simulink model "lab10_3"  (R2016a)
settings: Solver=VariableStepAuto  StartTime=0.0  StopTime=10.0  RelTol=1e-3
libraries: dspsrcs4 x1
settings Model: Creator=Student  LastModifiedBy=Student

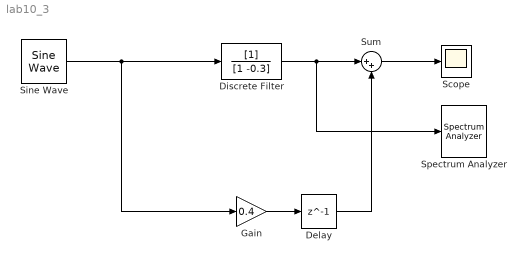
== system lab10_3 ==
  Delay : Delay  DelayLength=1  InitialCondition=0
  Discrete Filter : DiscreteFilter  Denominator=[1 -0.3]
  Gain : Gain  Gain=0.4
  Scope : Scope
  Sine Wave : dspsrcs4/Sine Wave  Amplitude=1  Frequency=100  Phase=0  SampleMode=Discrete  OutComplex=Real  CompMethod=Trigonometric fcn  TableSize=Speed  SampleTime=1/1000  SamplesPerFrame=1  ResetState=Restart at time zero  OutputFrames=off  dataType=double  wordLen=16  udDataType=sfix(16)  fracBitsMode=Best precision  numFracBits=15  OutDataTypeStr=double  LastOutDataTypeStr=double
  Spectrum Analyzer : SpectrumAnalyzer
  Sum : Sum  Inputs=|++
  wires:
  Sine Wave/1 -> Gain/1, Discrete Filter/1
  Gain/1 -> Delay/1
  Delay/1 -> Sum/2
  Discrete Filter/1 -> Spectrum Analyzer/1, Sum/1
  Sum/1 -> Scope/1
